simulink model "Part_E_Ramp_Simulink"  (R2018b)
settings: Solver=VariableStepAuto  StartTime=0.0  StopTime=t_dur  MaxStep=t_step  RelTol=1e-3
values from neighbouring files (symbols this model uses):
  b = 62    [Part_e_ramp.m]    (also in Part_e_step.m)
  gear = 9.73    [Part_e_ramp.m]    (also in Part_e_step.m)
  kb = 1.4e-4    (= 0.00014)    [Part_e_ramp.m]    (also in Part_e_step.m)
  l = 0.5    [Part_c.m]    (also in Part_d.m; Part_e_ramp.m; Part_e_step.m)
  La = 0.005    [Part_e_ramp.m]    (also in Part_e_step.m)
  Lf = 0.3    [Part_e_ramp.m]    (also in Part_e_step.m)
  m = 2110    [Part_e_ramp.m]    (also in Part_e_step.m)
  N = 126    [Part_c.m]    (also in Part_d.m; Part_e_ramp.m; Part_e_step.m)
  r = 1/6    (= 0.166666666667)    [Part_c.m]    (also in Part_d.m; Part_e_ramp.m; Part_e_step.m)
  Ra = 0.07    [Part_e_ramp.m]    (also in Part_e_step.m)
  Rf = 1.15    [Part_e_ramp.m]    (also in Part_e_step.m)
  rw = d / 2    (= 0.24)    [Part_e_ramp.m]    (also in Part_e_step.m)
  V = 100    [Part_e_ramp.m]    (also in Part_e_step.m = 250)
libraries: simulink x14
settings Model: Creator=carcione.6  LastModifiedBy=Nick Carcione

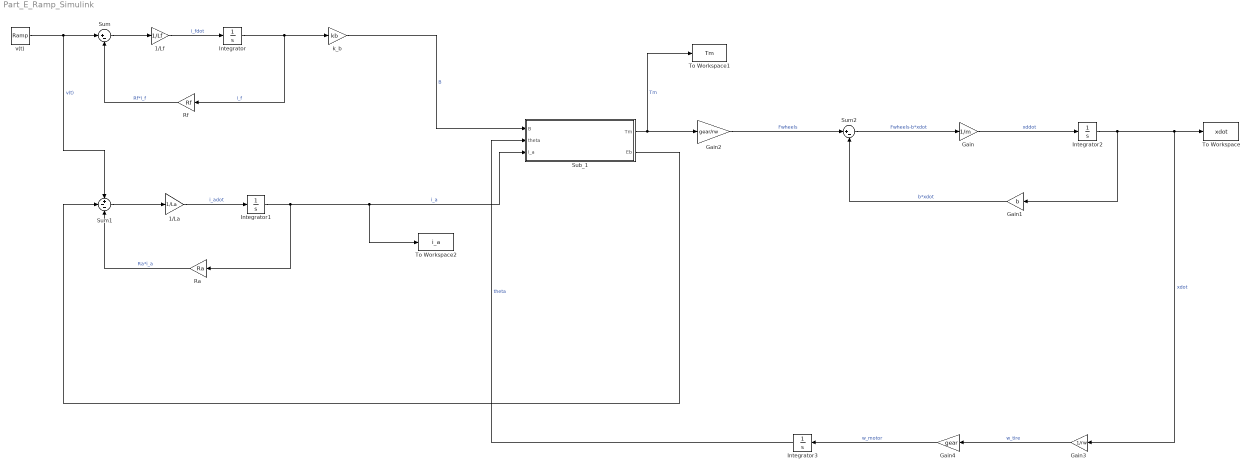
== system Part_E_Ramp_Simulink ==
  1/La : Gain  Gain=1/La
  1/Lf : Gain  Gain=1/Lf
  Gain : Gain  Gain=1/m
  Gain1 : Gain  Gain=b
  Gain2 : Gain  Gain=gear/rw
  Gain3 : Gain  Gain=1/rw
  Gain4 : Gain  Gain=gear
  Integrator{,1..3} (4 alike) : Integrator
  Ra : Gain  Gain=Ra
  Rf : Gain  Gain=Rf
  Sub_1 : Subsystem
  Sum : Sum  Inputs=|+-
  Sum1 : Sum  Inputs=+--
  Sum2 : Sum  Inputs=|+-
  To Workspace : ToWorkspace  VariableName=xdot  SaveFormat=Timeseries  SampleTime=-1
  To Workspace1 : ToWorkspace  VariableName=Tm  SaveFormat=Timeseries  SampleTime=-1
  To Workspace2 : ToWorkspace  VariableName=i_a  SaveFormat=Timeseries  SampleTime=-1
  k_b : Gain  Gain=kb
  v(t) : simulink/Sources/Ramp  slope=V  start=0  InitialOutput=0
  wires:
  Sub_1/1(Tm) -> To Workspace1/1, Gain2/1  "Tm"
  Integrator2/1 -> Gain3/1, To Workspace/1, Gain1/1  "xdot"
  Ra/1 -> Sum1/3  "Ra*i_a"
  Rf/1 -> Sum/2  "Rf*i_f"
  Gain3/1 -> Gain4/1  "w_tire"
  Integrator1/1 -> Ra/1, To Workspace2/1, Sub_1/3(i_a)  "i_a"
  Sum/1 -> 1/Lf/1
  v(t)/1 -> Sum1/1, Sum/1  "v(t)"
  k_b/1 -> Sub_1/1(B)  "B"
  Gain2/1 -> Sum2/1  "Fwheels"
  Gain/1 -> Integrator2/1  "xddot"
  Sub_1/2(Eb) -> Sum1/2
  Gain1/1 -> Sum2/2  "b*xdot"
  Integrator3/1 -> Sub_1/2(theta)  "theta"
  Gain4/1 -> Integrator3/1  "w_motor"
  Sum1/1 -> 1/La/1
  1/Lf/1 -> Integrator/1  "i_fdot"
  Integrator/1 -> Rf/1, k_b/1  "i_f"
  1/La/1 -> Integrator1/1  "i_adot"
  Sum2/1 -> Gain/1  "Fwheels-b*xdot"

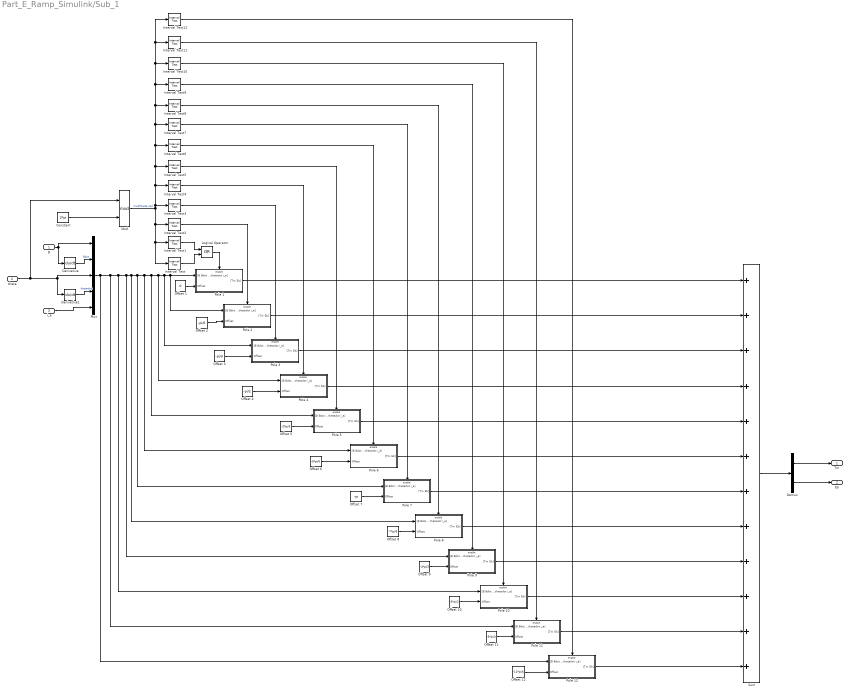
== system Part_E_Ramp_Simulink/Sub_1 ==
  B : Inport
  theta : Inport  Port=2
  i_a : Inport  Port=3
  Constant : Constant  Value=2*pi
  Demux : Demux  Outputs=2
  Derivative : Derivative
  Derivative1 : Derivative
  Interval Test : simulink/Logic and Bit Operations/Interval Test  IntervalClosedRight=off  uplimit=2*pi  IntervalClosedLeft=on  lowlimit=23*pi/12  OutDataTypeStr=boolean
  Interval Test1 : simulink/Logic and Bit Operations/Interval Test  IntervalClosedRight=off  uplimit=pi/12  IntervalClosedLeft=on  lowlimit=0  OutDataTypeStr=boolean
  Interval Test10 : simulink/Logic and Bit Operations/Interval Test  IntervalClosedRight=off  uplimit=19*pi/12  IntervalClosedLeft=on  lowlimit=17*pi/12  OutDataTypeStr=boolean
  Interval Test11 : simulink/Logic and Bit Operations/Interval Test  IntervalClosedRight=off  uplimit=21*pi/12  IntervalClosedLeft=on  lowlimit=19*pi/12  OutDataTypeStr=boolean
  Interval Test12 : simulink/Logic and Bit Operations/Interval Test  IntervalClosedRight=off  uplimit=23*pi/12  IntervalClosedLeft=on  lowlimit=21*pi/12  OutDataTypeStr=boolean
  Interval Test2 : simulink/Logic and Bit Operations/Interval Test  IntervalClosedRight=off  uplimit=3*pi/12  IntervalClosedLeft=on  lowlimit=pi/12  OutDataTypeStr=boolean
  Interval Test3 : simulink/Logic and Bit Operations/Interval Test  IntervalClosedRight=off  uplimit=5*pi/12  IntervalClosedLeft=on  lowlimit=3*pi/12  OutDataTypeStr=boolean
  Interval Test4 : simulink/Logic and Bit Operations/Interval Test  IntervalClosedRight=off  uplimit=7*pi/12  IntervalClosedLeft=on  lowlimit=5*pi/12  OutDataTypeStr=boolean
  Interval Test5 : simulink/Logic and Bit Operations/Interval Test  IntervalClosedRight=off  uplimit=9*pi/12  IntervalClosedLeft=on  lowlimit=7*pi/12  OutDataTypeStr=boolean
  Interval Test6 : simulink/Logic and Bit Operations/Interval Test  IntervalClosedRight=off  uplimit=11*pi/12  IntervalClosedLeft=on  lowlimit=9*pi/12  OutDataTypeStr=boolean
  Interval Test7 : simulink/Logic and Bit Operations/Interval Test  IntervalClosedRight=off  uplimit=13*pi/12  IntervalClosedLeft=on  lowlimit=11*pi/12  OutDataTypeStr=boolean
  Interval Test8 : simulink/Logic and Bit Operations/Interval Test  IntervalClosedRight=off  uplimit=15*pi/12  IntervalClosedLeft=on  lowlimit=13*pi/12  OutDataTypeStr=boolean
  Interval Test9 : simulink/Logic and Bit Operations/Interval Test  IntervalClosedRight=off  uplimit=17*pi/12  IntervalClosedLeft=on  lowlimit=15*pi/12  OutDataTypeStr=boolean
  Logical Operator : Logic  Operator=OR  AllPortsSameDT=off  OutDataTypeStr=boolean
  Mod : Math  Operator=mod  SaturateOnIntegerOverflow=on
  Mux : Mux  Inputs=5
  Offset 1 : Constant  Value=0
  Offset 10 : Constant  Value=-3*pi/2
  Offset 11 : Constant  Value=-5*pi/3
  Offset 12 : Constant  Value=-11*pi/6
  Offset 2 : Constant  Value=-pi/6
  Offset 3 : Constant  Value=-pi/3
  Offset 4 : Constant  Value=-pi/2
  Offset 5 : Constant  Value=-2*pi/3
  Offset 6 : Constant  Value=-5*pi/6
  Offset 7 : Constant  Value=-pi
  Offset 8 : Constant  Value=-7*pi/6
  Offset 9 : Constant  Value=-4*pi/3
  Pole 1 : Subsystem
  Pole 10 : Subsystem
  Pole 11 : Subsystem
  Pole 12 : Subsystem
  Pole 2 : Subsystem
  Pole 3 : Subsystem
  Pole 4 : Subsystem
  Pole 5 : Subsystem
  Pole 6 : Subsystem
  Pole 7 : Subsystem
  Pole 8 : Subsystem
  Pole 9 : Subsystem
  Sum : Sum  Inputs=++++++++++++
  Tm : Outport
  Eb : Outport  Port=2
  wires:
  i_a/1 -> Mux/5
  B/1 -> Derivative/1, Mux/1
  Derivative/1 -> Mux/2  "Bdot"
  Derivative1/1 -> Mux/4  "thetadot"
  theta/1 -> Mod/1, Derivative1/1, Mux/3
  Offset 1/1 -> Pole 1/2(Offset)
  Offset 2/1 -> Pole 2/2(Offset)
  Offset 3/1 -> Pole 3/2(Offset)
  Offset 4/1 -> Pole 4/2(Offset)
  Mux/1 -> Pole 12/1("[B Bdot theta thetadot i_a]"), Pole 11/1("[B Bdot theta thetadot i_a]"), Pole 10/1("[B Bdot theta thetadot i_a]"), Pole 9/1("[B Bdot theta thetadot i_a]"), Pole 8/1("[B Bdot theta thetadot i_a]"), Pole 7/1("[B Bdot theta thetadot i_a]"), Pole 6/1("[B Bdot theta thetadot i_a]"), Pole 5/1("[B Bdot theta thetadot i_a]"), Pole 4/1("[B Bdot theta thetadot i_a]"), Pole 3/1("[B Bdot theta thetadot i_a]"), Pole 2/1("[B Bdot theta thetadot i_a]"), Pole 1/1("[B Bdot theta thetadot i_a]")
  Constant/1 -> Mod/2
  Mod/1 -> Interval Test2/1, Interval Test/1, Interval Test1/1, Interval Test6/1, Interval Test7/1, Interval Test9/1, Interval Test10/1, Interval Test11/1, Interval Test12/1, Interval Test8/1, Interval Test5/1, Interval Test4/1, Interval Test3/1  "mod(theta,2pi)"
  Interval Test1/1 -> Logical Operator/1
  Interval Test/1 -> Logical Operator/2
  Logical Operator/1 -> Pole 1/Enable
  Interval Test2/1 -> Pole 2/Enable
  Interval Test3/1 -> Pole 3/Enable
  Interval Test4/1 -> Pole 4/Enable
  Pole 1/1("[Tm Eb]") -> Sum/1
  Pole 4/1("[Tm Eb]") -> Sum/4
  Pole 3/1("[Tm Eb]") -> Sum/3
  Pole 2/1("[Tm Eb]") -> Sum/2
  Sum/1 -> Demux/1
  Demux/1 -> Tm/1
  Demux/2 -> Eb/1
  Interval Test5/1 -> Pole 5/Enable
  Interval Test6/1 -> Pole 6/Enable
  Interval Test7/1 -> Pole 7/Enable
  Interval Test8/1 -> Pole 8/Enable
  Interval Test9/1 -> Pole 9/Enable
  Interval Test10/1 -> Pole 10/Enable
  Interval Test11/1 -> Pole 11/Enable
  Interval Test12/1 -> Pole 12/Enable
  Pole 12/1("[Tm Eb]") -> Sum/12
  Pole 11/1("[Tm Eb]") -> Sum/11
  Pole 10/1("[Tm Eb]") -> Sum/10
  Pole 9/1("[Tm Eb]") -> Sum/9
  Pole 8/1("[Tm Eb]") -> Sum/8
  Pole 7/1("[Tm Eb]") -> Sum/7
  Pole 6/1("[Tm Eb]") -> Sum/6
  Pole 5/1("[Tm Eb]") -> Sum/5
  Offset 12/1 -> Pole 12/2(Offset)
  Offset 11/1 -> Pole 11/2(Offset)
  Offset 10/1 -> Pole 10/2(Offset)
  Offset 9/1 -> Pole 9/2(Offset)
  Offset 8/1 -> Pole 8/2(Offset)
  Offset 7/1 -> Pole 7/2(Offset)
  Offset 6/1 -> Pole 6/2(Offset)
  Offset 5/1 -> Pole 5/2(Offset)

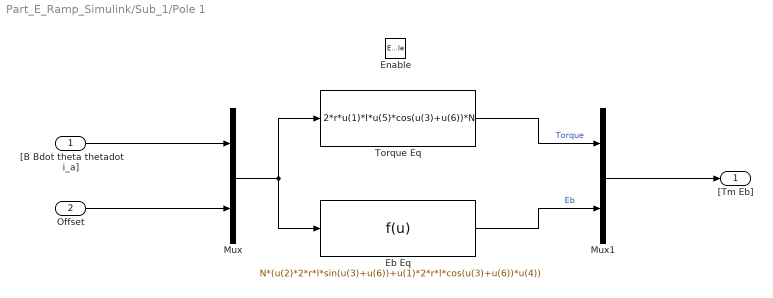
== system Part_E_Ramp_Simulink/Sub_1/Pole 1 ==
  "[B Bdot theta thetadot i_a]" : Inport
  Offset : Inport  Port=2
  Enable : EnablePort
  Eb Eq : Fcn  Expr=N*(u(2)*2*r*l*sin(u(3)+u(6))+u(1)*2*r*l*cos(u(3)+u(6))*u(4))
  Mux : Mux  Inputs=2
  Mux1 : Mux  Inputs=2
  Torque Eq : Fcn  Expr=2*r*u(1)*l*u(5)*cos(u(3)+u(6))*N
  "[Tm Eb]" : Outport  OutputWhenDisabled=reset  InitialOutput=[0,0]
  wires:
  "[B Bdot theta thetadot i_a]"/1 -> Mux/1
  Offset/1 -> Mux/2
  Mux/1 -> Eb Eq/1, Torque Eq/1
  Torque Eq/1 -> Mux1/1  "Torque"
  Eb Eq/1 -> Mux1/2  "Eb"
  Mux1/1 -> "[Tm Eb]"/1

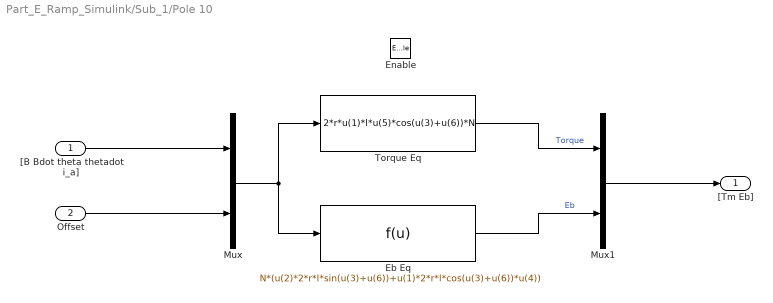
== system Part_E_Ramp_Simulink/Sub_1/Pole 10 ==
  "[B Bdot theta thetadot i_a]" : Inport
  Offset : Inport  Port=2
  Enable : EnablePort
  Eb Eq : Fcn  Expr=N*(u(2)*2*r*l*sin(u(3)+u(6))+u(1)*2*r*l*cos(u(3)+u(6))*u(4))
  Mux : Mux  Inputs=2
  Mux1 : Mux  Inputs=2
  Torque Eq : Fcn  Expr=2*r*u(1)*l*u(5)*cos(u(3)+u(6))*N
  "[Tm Eb]" : Outport  OutputWhenDisabled=reset  InitialOutput=[0,0]
  wires:
  Mux1/1 -> "[Tm Eb]"/1
  Eb Eq/1 -> Mux1/2  "Eb"
  Torque Eq/1 -> Mux1/1  "Torque"
  Mux/1 -> Torque Eq/1, Eb Eq/1
  Offset/1 -> Mux/2
  "[B Bdot theta thetadot i_a]"/1 -> Mux/1

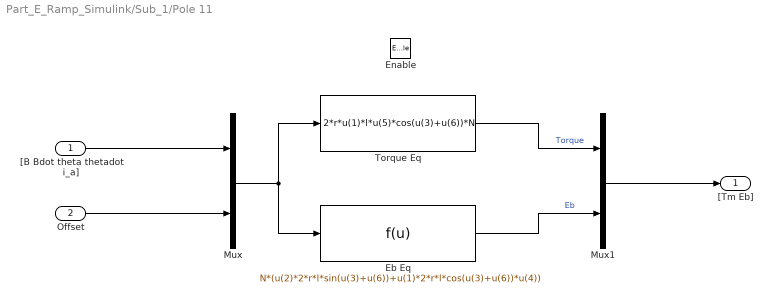
== system Part_E_Ramp_Simulink/Sub_1/Pole 11 ==
  "[B Bdot theta thetadot i_a]" : Inport
  Offset : Inport  Port=2
  Enable : EnablePort
  Eb Eq : Fcn  Expr=N*(u(2)*2*r*l*sin(u(3)+u(6))+u(1)*2*r*l*cos(u(3)+u(6))*u(4))
  Mux : Mux  Inputs=2
  Mux1 : Mux  Inputs=2
  Torque Eq : Fcn  Expr=2*r*u(1)*l*u(5)*cos(u(3)+u(6))*N
  "[Tm Eb]" : Outport  OutputWhenDisabled=reset  InitialOutput=[0,0]
  wires:
  "[B Bdot theta thetadot i_a]"/1 -> Mux/1
  Offset/1 -> Mux/2
  Mux/1 -> Eb Eq/1, Torque Eq/1
  Torque Eq/1 -> Mux1/1  "Torque"
  Eb Eq/1 -> Mux1/2  "Eb"
  Mux1/1 -> "[Tm Eb]"/1

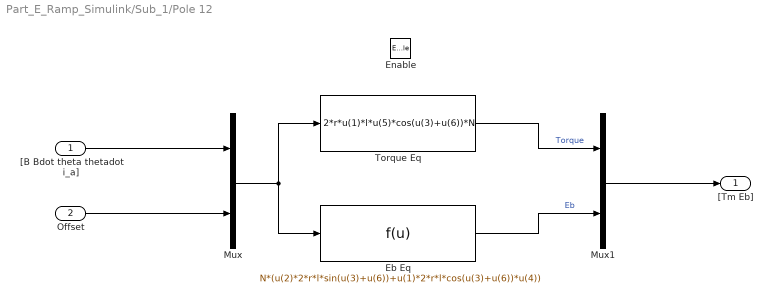
== system Part_E_Ramp_Simulink/Sub_1/Pole 12 ==
  "[B Bdot theta thetadot i_a]" : Inport
  Offset : Inport  Port=2
  Enable : EnablePort
  Eb Eq : Fcn  Expr=N*(u(2)*2*r*l*sin(u(3)+u(6))+u(1)*2*r*l*cos(u(3)+u(6))*u(4))
  Mux : Mux  Inputs=2
  Mux1 : Mux  Inputs=2
  Torque Eq : Fcn  Expr=2*r*u(1)*l*u(5)*cos(u(3)+u(6))*N
  "[Tm Eb]" : Outport  OutputWhenDisabled=reset  InitialOutput=[0,0]
  wires:
  Mux1/1 -> "[Tm Eb]"/1
  Eb Eq/1 -> Mux1/2  "Eb"
  Torque Eq/1 -> Mux1/1  "Torque"
  Mux/1 -> Torque Eq/1, Eb Eq/1
  Offset/1 -> Mux/2
  "[B Bdot theta thetadot i_a]"/1 -> Mux/1

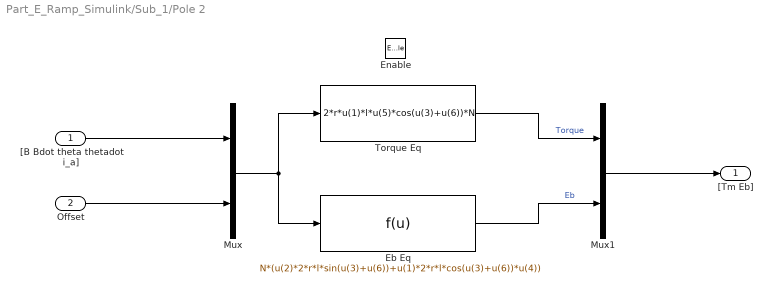
== system Part_E_Ramp_Simulink/Sub_1/Pole 2 ==
  "[B Bdot theta thetadot i_a]" : Inport
  Offset : Inport  Port=2
  Enable : EnablePort
  Eb Eq : Fcn  Expr=N*(u(2)*2*r*l*sin(u(3)+u(6))+u(1)*2*r*l*cos(u(3)+u(6))*u(4))
  Mux : Mux  Inputs=2
  Mux1 : Mux  Inputs=2
  Torque Eq : Fcn  Expr=2*r*u(1)*l*u(5)*cos(u(3)+u(6))*N
  "[Tm Eb]" : Outport  OutputWhenDisabled=reset  InitialOutput=[0,0]
  wires:
  Mux1/1 -> "[Tm Eb]"/1
  Eb Eq/1 -> Mux1/2  "Eb"
  Torque Eq/1 -> Mux1/1  "Torque"
  Mux/1 -> Torque Eq/1, Eb Eq/1
  Offset/1 -> Mux/2
  "[B Bdot theta thetadot i_a]"/1 -> Mux/1

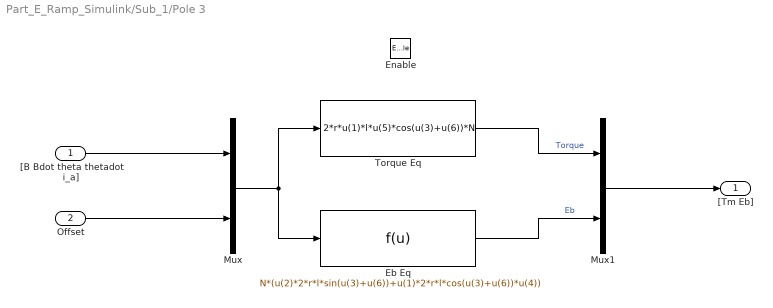
== system Part_E_Ramp_Simulink/Sub_1/Pole 3 ==
  "[B Bdot theta thetadot i_a]" : Inport
  Offset : Inport  Port=2
  Enable : EnablePort
  Eb Eq : Fcn  Expr=N*(u(2)*2*r*l*sin(u(3)+u(6))+u(1)*2*r*l*cos(u(3)+u(6))*u(4))
  Mux : Mux  Inputs=2
  Mux1 : Mux  Inputs=2
  Torque Eq : Fcn  Expr=2*r*u(1)*l*u(5)*cos(u(3)+u(6))*N
  "[Tm Eb]" : Outport  OutputWhenDisabled=reset  InitialOutput=[0,0]
  wires:
  "[B Bdot theta thetadot i_a]"/1 -> Mux/1
  Offset/1 -> Mux/2
  Mux/1 -> Eb Eq/1, Torque Eq/1
  Torque Eq/1 -> Mux1/1  "Torque"
  Eb Eq/1 -> Mux1/2  "Eb"
  Mux1/1 -> "[Tm Eb]"/1

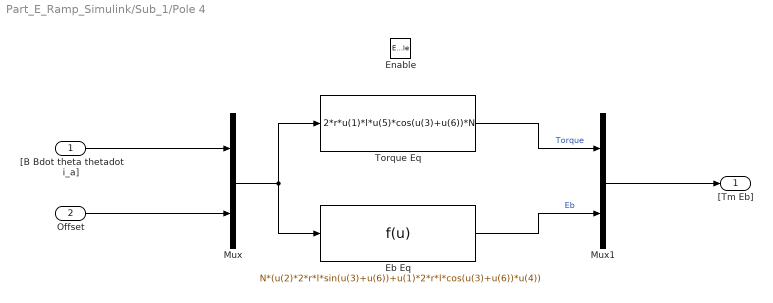
== system Part_E_Ramp_Simulink/Sub_1/Pole 4 ==
  "[B Bdot theta thetadot i_a]" : Inport
  Offset : Inport  Port=2
  Enable : EnablePort
  Eb Eq : Fcn  Expr=N*(u(2)*2*r*l*sin(u(3)+u(6))+u(1)*2*r*l*cos(u(3)+u(6))*u(4))
  Mux : Mux  Inputs=2
  Mux1 : Mux  Inputs=2
  Torque Eq : Fcn  Expr=2*r*u(1)*l*u(5)*cos(u(3)+u(6))*N
  "[Tm Eb]" : Outport  OutputWhenDisabled=reset  InitialOutput=[0,0]
  wires:
  Mux1/1 -> "[Tm Eb]"/1
  Eb Eq/1 -> Mux1/2  "Eb"
  Torque Eq/1 -> Mux1/1  "Torque"
  Mux/1 -> Torque Eq/1, Eb Eq/1
  Offset/1 -> Mux/2
  "[B Bdot theta thetadot i_a]"/1 -> Mux/1

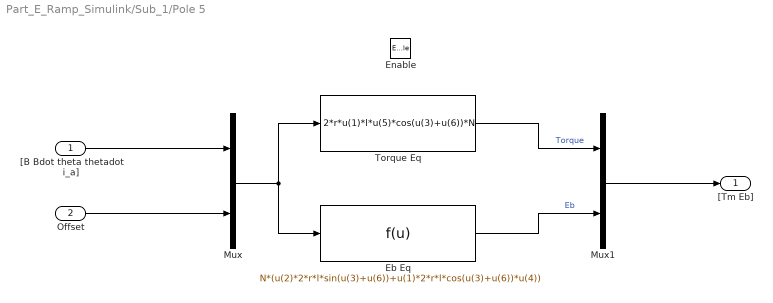
== system Part_E_Ramp_Simulink/Sub_1/Pole 5 ==
  "[B Bdot theta thetadot i_a]" : Inport
  Offset : Inport  Port=2
  Enable : EnablePort
  Eb Eq : Fcn  Expr=N*(u(2)*2*r*l*sin(u(3)+u(6))+u(1)*2*r*l*cos(u(3)+u(6))*u(4))
  Mux : Mux  Inputs=2
  Mux1 : Mux  Inputs=2
  Torque Eq : Fcn  Expr=2*r*u(1)*l*u(5)*cos(u(3)+u(6))*N
  "[Tm Eb]" : Outport  OutputWhenDisabled=reset  InitialOutput=[0,0]
  wires:
  "[B Bdot theta thetadot i_a]"/1 -> Mux/1
  Offset/1 -> Mux/2
  Mux/1 -> Eb Eq/1, Torque Eq/1
  Torque Eq/1 -> Mux1/1  "Torque"
  Eb Eq/1 -> Mux1/2  "Eb"
  Mux1/1 -> "[Tm Eb]"/1

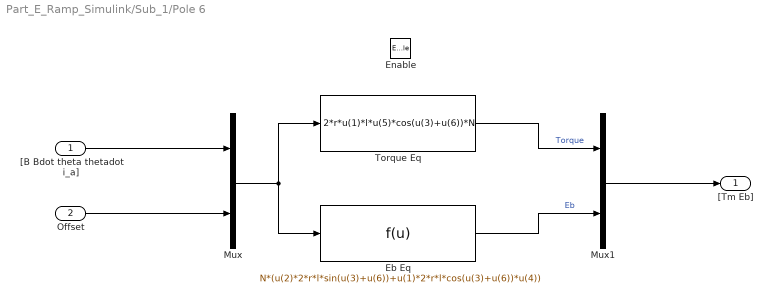
== system Part_E_Ramp_Simulink/Sub_1/Pole 6 ==
  "[B Bdot theta thetadot i_a]" : Inport
  Offset : Inport  Port=2
  Enable : EnablePort
  Eb Eq : Fcn  Expr=N*(u(2)*2*r*l*sin(u(3)+u(6))+u(1)*2*r*l*cos(u(3)+u(6))*u(4))
  Mux : Mux  Inputs=2
  Mux1 : Mux  Inputs=2
  Torque Eq : Fcn  Expr=2*r*u(1)*l*u(5)*cos(u(3)+u(6))*N
  "[Tm Eb]" : Outport  OutputWhenDisabled=reset  InitialOutput=[0,0]
  wires:
  Mux1/1 -> "[Tm Eb]"/1
  Eb Eq/1 -> Mux1/2  "Eb"
  Torque Eq/1 -> Mux1/1  "Torque"
  Mux/1 -> Torque Eq/1, Eb Eq/1
  Offset/1 -> Mux/2
  "[B Bdot theta thetadot i_a]"/1 -> Mux/1

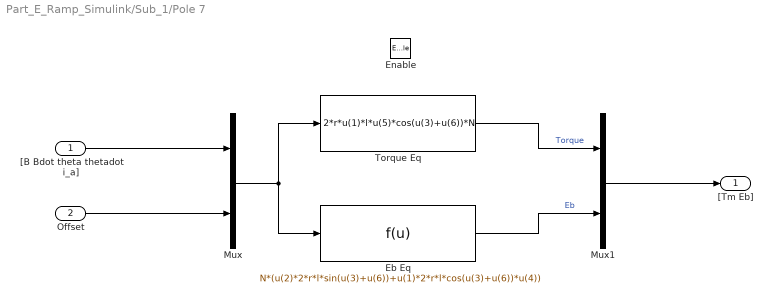
== system Part_E_Ramp_Simulink/Sub_1/Pole 7 ==
  "[B Bdot theta thetadot i_a]" : Inport
  Offset : Inport  Port=2
  Enable : EnablePort
  Eb Eq : Fcn  Expr=N*(u(2)*2*r*l*sin(u(3)+u(6))+u(1)*2*r*l*cos(u(3)+u(6))*u(4))
  Mux : Mux  Inputs=2
  Mux1 : Mux  Inputs=2
  Torque Eq : Fcn  Expr=2*r*u(1)*l*u(5)*cos(u(3)+u(6))*N
  "[Tm Eb]" : Outport  OutputWhenDisabled=reset  InitialOutput=[0,0]
  wires:
  "[B Bdot theta thetadot i_a]"/1 -> Mux/1
  Offset/1 -> Mux/2
  Mux/1 -> Eb Eq/1, Torque Eq/1
  Torque Eq/1 -> Mux1/1  "Torque"
  Eb Eq/1 -> Mux1/2  "Eb"
  Mux1/1 -> "[Tm Eb]"/1

== system Part_E_Ramp_Simulink/Sub_1/Pole 8 ==
  "[B Bdot theta thetadot i_a]" : Inport
  Offset : Inport  Port=2
  Enable : EnablePort
  Eb Eq : Fcn  Expr=N*(u(2)*2*r*l*sin(u(3)+u(6))+u(1)*2*r*l*cos(u(3)+u(6))*u(4))
  Mux : Mux  Inputs=2
  Mux1 : Mux  Inputs=2
  Torque Eq : Fcn  Expr=2*r*u(1)*l*u(5)*cos(u(3)+u(6))*N
  "[Tm Eb]" : Outport  OutputWhenDisabled=reset  InitialOutput=[0,0]
  wires:
  Mux1/1 -> "[Tm Eb]"/1
  Eb Eq/1 -> Mux1/2  "Eb"
  Torque Eq/1 -> Mux1/1  "Torque"
  Mux/1 -> Torque Eq/1, Eb Eq/1
  Offset/1 -> Mux/2
  "[B Bdot theta thetadot i_a]"/1 -> Mux/1

== system Part_E_Ramp_Simulink/Sub_1/Pole 9 ==
  "[B Bdot theta thetadot i_a]" : Inport
  Offset : Inport  Port=2
  Enable : EnablePort
  Eb Eq : Fcn  Expr=N*(u(2)*2*r*l*sin(u(3)+u(6))+u(1)*2*r*l*cos(u(3)+u(6))*u(4))
  Mux : Mux  Inputs=2
  Mux1 : Mux  Inputs=2
  Torque Eq : Fcn  Expr=2*r*u(1)*l*u(5)*cos(u(3)+u(6))*N
  "[Tm Eb]" : Outport  OutputWhenDisabled=reset  InitialOutput=[0,0]
  wires:
  "[B Bdot theta thetadot i_a]"/1 -> Mux/1
  Offset/1 -> Mux/2
  Mux/1 -> Eb Eq/1, Torque Eq/1
  Torque Eq/1 -> Mux1/1  "Torque"
  Eb Eq/1 -> Mux1/2  "Eb"
  Mux1/1 -> "[Tm Eb]"/1
